simulink model "Project_2_2020a"  (R2020a)
settings: Solver=ode15s  StartTime=0.0  StopTime=10  MaxStep=0.2  RelTol=1e-2  EnableMultiTasking=on
model workspace (MAT data in the model file):
  g_density = 5
values from neighbouring files (symbols this model uses):
  Aa = 0    [execute_model_2020a.m]
  Ab = 0    [execute_model_2020a.m]
  Ac = 0    [execute_model_2020a.m]
  Ax = 0    [execute_model_2020a.m]
  Ay = 0    [execute_model_2020a.m]
  Az = 0    [execute_model_2020a.m]
  B = [24.233423136094 6.1219332628706 -6.1219332628706 -24.233423136094 -18.111489873223 18.111489873223 ... (first row only)    [execute_model_2020a.m]
  flange_len = 3    [execute_model_2020a.m]
  flange_thick = 0.8    [execute_model_2020a.m]
  flange_width = 2.25    [execute_model_2020a.m]
  hex_skew = -0.25    [execute_model_2020a.m]
  ka = 0    [execute_model_2020a.m]
  kb = 0    [execute_model_2020a.m]
  kc = 0    [execute_model_2020a.m]
  Kd = 8    [execute_model_2020a.m]
  Ki = 11.5    [execute_model_2020a.m]
  Kp = 450    [execute_model_2020a.m]
  kx = 0    [execute_model_2020a.m]
  ky = 0    [execute_model_2020a.m]
  kz = 75    [execute_model_2020a.m]
  leg_rad = 3    [execute_model_2020a.m]
  nom_length = 30    [execute_model_2020a.m]
  P = [14.574164873203 11.040422061358 -11.040422061358 -14.574164873203 -3.5337428118454 3.5337428118454 ... (first row only)    [execute_model_2020a.m]
  pa = 0    [execute_model_2020a.m]
  pb = 0    [execute_model_2020a.m]
  pc = 0    [execute_model_2020a.m]
  platform_rad = 18    [execute_model_2020a.m]
  platform_thick = 2    [execute_model_2020a.m]
  px = 0    [execute_model_2020a.m]
  py = 0    [execute_model_2020a.m]
  pz = 0    [execute_model_2020a.m]
  wa = 0    [execute_model_2020a.m]
  wb = 0    [execute_model_2020a.m]
  wc = 0    [execute_model_2020a.m]
  wx = 0    [execute_model_2020a.m]
  wy = 0    [execute_model_2020a.m]
  wz = 0    [execute_model_2020a.m]
undefined symbols (not defined in the file or in its folder): X, Y, Z
libraries: sm_stewart_platform_lib x13, sm_lib x10, nesl_utility x8, simulink x2, Parts_Lib x1, Contact_Forces_Lib x1, simulink_extras x1
(part 2 of 2)

== system Project_2_2020a/dy ==
  t : Inport
  Add : Sum  Inputs=|++
  Add2 : Sum  Inputs=++|
  amp1 : Gain  Gain=A
  amp2 : Gain  Gain=w*A*pi/180
  deg2rad : Gain  Gain=pi/180
  freq : Gain  Gain=w
  offset : Constant  Value=k  VectorParams1D=off
  phase : Constant  Value=p  VectorParams1D=off
  sin cos : Trigonometry  Operator=sincos
  f : Outport  VectorParamsAs1DForOutWhenUnconnected=off
  f' : Outport  Port=2  VectorParamsAs1DForOutWhenUnconnected=off
  wires:
  t/1 -> freq/1
  Add/1 -> deg2rad/1
  phase/1 -> Add/2
  amp2/1 -> f'/1
  Add2/1 -> f/1
  offset/1 -> Add2/1
  sin cos/1 -> amp1/1
  sin cos/2 -> amp2/1
  amp1/1 -> Add2/2
  freq/1 -> Add/1
  deg2rad/1 -> sin cos/1

== system Project_2_2020a/dz ==
  t : Inport
  Add : Sum  Inputs=|++
  Add2 : Sum  Inputs=++|
  amp1 : Gain  Gain=A
  amp2 : Gain  Gain=w*A*pi/180
  deg2rad : Gain  Gain=pi/180
  freq : Gain  Gain=w
  offset : Constant  Value=k  VectorParams1D=off
  phase : Constant  Value=p  VectorParams1D=off
  sin cos : Trigonometry  Operator=sincos
  f : Outport  VectorParamsAs1DForOutWhenUnconnected=off
  f' : Outport  Port=2  VectorParamsAs1DForOutWhenUnconnected=off
  wires:
  t/1 -> freq/1
  Add/1 -> deg2rad/1
  phase/1 -> Add/2
  amp2/1 -> f'/1
  Add2/1 -> f/1
  offset/1 -> Add2/1
  sin cos/1 -> amp1/1
  sin cos/2 -> amp2/1
  amp1/1 -> Add2/2
  freq/1 -> Add/1
  deg2rad/1 -> sin cos/1

== system Project_2_2020a/Euler XYZ Derivative/Skew Op ==
  v : Inport
  Demux : Demux  Outputs=3
  Demux1 : Demux  Outputs=3
  Gain : Gain  Gain=-1
  Mux6 : Mux  Inputs=9
  Reshape 9x1->3x3 : Reshape  OutputDimensionality=Customize  OutputDimensions=[3,3]
  Zero : Constant  Value=0
  v~ : Outport  VectorParamsAs1DForOutWhenUnconnected=off
  wires:
  Mux6/1 -> Reshape 9x1->3x3/1
  v/1 -> Demux/1, Gain/1
  Gain/1 -> Demux1/1
  Reshape 9x1->3x3/1 -> v~/1
  Zero/1 -> Mux6/1, Mux6/5, Mux6/9
  Demux/3 -> Mux6/2
  Demux1/2 -> Mux6/3
  Demux1/3 -> Mux6/4
  Demux/1 -> Mux6/6
  Demux/2 -> Mux6/7
  Demux1/1 -> Mux6/8

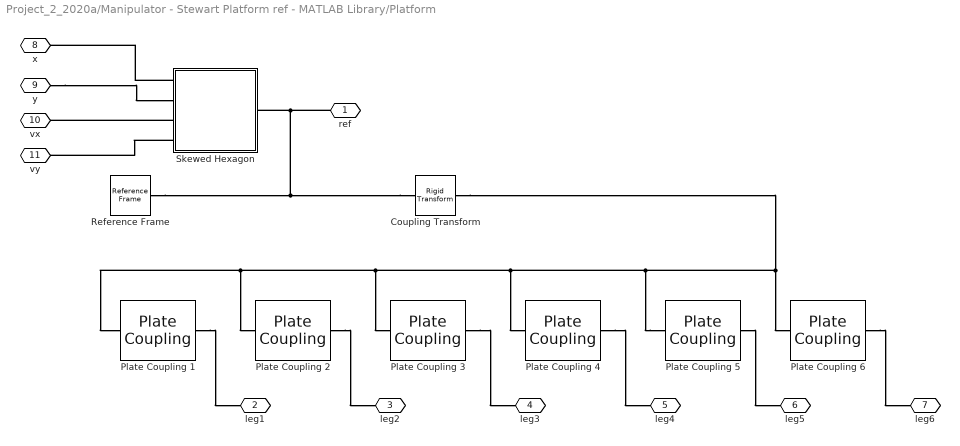
== system Project_2_2020a/Manipulator - Stewart Platform ref - MATLAB Library/Platform ==
  Coupling Transform : sm_lib/Frames and Transforms/Rigid Transform  TranslationMethod=StandardAxis  TranslationStandardOffset=(1 - 2 * kind_val) * (hex_thick / 2 + flange_len)  TranslationLengthUnit=cm  TranslationStandardAxis=+Z  TranslationCartesianOffset=[0 0 0]  TranslationROffset=0  TranslationROffsetUnits=m  TranslationZOffset=0  TranslationZOffsetUnits=m  TranslationThetaOffset=0  TranslationThetaOffsetUnits=deg  RotationMethod=AlignedAxes  RotationAngleUnits=deg  RotationStandardAxis=+Z  RotationAngle=0  RotationArbitraryAxis=[0 0 1]  FollAlignAxisA=+Z  BaseAlignAxisA=+X  FollAlignAxisB=+X  BaseAlignAxisB=+Z  RotationSequenceAxes=FollowerAxes  RotationSequence=XYX  RotationSequenceAngles=[0 0 0]  RotationSequenceAnglesUnits=deg  RotationMatrix=[1 0 0; 0 1 0; 0 0 1]  Quaternion=[1 0 0 0]
  Plate Coupling 1 : sm_stewart_platform_lib/Plate Coupling  index=0 + kind_val  hex_rad=hex_rad  hex_skew=hex_skew  flange_width=flange_width  flange_thick=flange_thick  flange_sep=flange_sep  flange_ref_rot=kind_val * 180
  Plate Coupling 2 : sm_stewart_platform_lib/Plate Coupling  index=1 + kind_val  hex_rad=hex_rad  hex_skew=hex_skew  flange_width=flange_width  flange_thick=flange_thick  flange_sep=flange_sep  flange_ref_rot=kind_val * 180
  Plate Coupling 3 : sm_stewart_platform_lib/Plate Coupling  index=2 + kind_val  hex_rad=hex_rad  hex_skew=hex_skew  flange_width=flange_width  flange_thick=flange_thick  flange_sep=flange_sep  flange_ref_rot=kind_val * 180
  Plate Coupling 4 : sm_stewart_platform_lib/Plate Coupling  index=3 + kind_val  hex_rad=hex_rad  hex_skew=hex_skew  flange_width=flange_width  flange_thick=flange_thick  flange_sep=flange_sep  flange_ref_rot=kind_val * 180
  Plate Coupling 5 : sm_stewart_platform_lib/Plate Coupling  index=4 + kind_val  hex_rad=hex_rad  hex_skew=hex_skew  flange_width=flange_width  flange_thick=flange_thick  flange_sep=flange_sep  flange_ref_rot=kind_val * 180
  Plate Coupling 6 : sm_stewart_platform_lib/Plate Coupling  index=mod(5 + kind_val, 6)  hex_rad=hex_rad  hex_skew=hex_skew  flange_width=flange_width  flange_thick=flange_thick  flange_sep=flange_sep  flange_ref_rot=kind_val * 180
  Reference Frame : sm_lib/Frames and Transforms/Reference Frame
  Skewed Hexagon : Subsystem  mask(Skewed Hexagon){rad=hex_rad, thick=hex_thick, skew=hex_skew, diffuse=diffuse, specualr=specular, shininess=shininess}
      mask prompts: rad "Radius (cm)"; thick "Thickness (cm)"; diffuse "Diffuse (rgba)"; specualr "Specular (rgba)"; shininess "Shininess (0-128)"
      mask help:
      | Models a hexagonal prism with 3-fold symmetry.
      |
      | A skew factor in the range (-0.5, +0.5) controls the shape of the hexagon.  A zero skew factor produces a regular hexagon cross section, and values toward +/- 0.5 produce progressively more triangular hexagons.
      mask init:
      | angles = pi/3 * ((0:1:5) + skew * [+1 -1 +1 -1 +1 -1]);
      | cross_sect = rad * [cos(angles); sin(angles)]';
      mask Help:
      | A <em>Skewed Hexagon</em> models a hexagonal prism with 3-fold symmetry.
      | 
      | A skew factor in the range (-0.5, +0.5) controls the shape of the hexagon.  A zero
      | skew factor produces a regular hexagon cross section, and values toward +/- 0.5
      | produce progressively more triangular hexagons.
      | 
      | See <em>Skewed Hexagons</em> in the documentation of the <em>Hexagon Plate</em>
      | block for more details.
      | 
      | <h3>Geometry</h3>
      | 
      | The <em>Geom</em> tab parameters specify the geometry of the skewed hexagon.
      | 
      | <ul>
      | 
      | <li> <b>Radius</b> The radius of thee circle on which the vertices of
      |   the hexagonal cross section lie.
      | 
      | <li> <b> Thickness</b> The thickness (length) of the hexagonal prism.
      | 
      | <li> <b>Skew</b> The skew factor of the hexagonal cross section, in the
      |   range (-0.5, +0.5).
      | 
      | </ul>
      | 
      | <h3>Visualization</h3>
      | 
      | The <em>Graphics</em> tab parameters specify the visualization aspects of the skewed
      | hexagon.
      | 
      | 
      | <ul>
      | 
      | <li> <b>Diffuse</b> The diffuse color of the skewed hexagon.  This is an RGB
      | 3-vector or an RGBA 4-vector with all components in the range [0, 1].
      | 
      | <li> <b>Specular</b> The specular color of the skewed hexagon.  This is an RGB
      | 3-vector or an RGBA 4-vector with all components in the range [0, 1].
      | 
      | <li> <b>Shininess</b> The shininess of the skewed hexagon.  This is a scalar
      | value in the range [0, 128].
      | 
      | </ul>
      | 
      | 
      | <h3>Ports</h3>
      | 
      | <ul>
      | 
      | <li> <b>ref</b> Reference frame of the skewed hexagon.  The origin of this frame
      |   is located at the center of the hexagonal prism, and the z-axis is aligned
      |   with the axis of the prism.
      | 
      | </ul>
      mask Display:
      | image('sm_stewart_platform_skewedhexagon.png')
      | color('white')
      | port_label('RConn', 1, 'ref')
  ref : PMIOPort  Side=Left
  leg1 : PMIOPort  Port=2  Side=Right
  leg2 : PMIOPort  Port=3  Side=Right
  leg3 : PMIOPort  Port=4  Side=Right
  leg4 : PMIOPort  Port=5  Side=Right
  leg5 : PMIOPort  Port=6  Side=Right
  leg6 : PMIOPort  Port=7  Side=Right
  x : PMIOPort  Port=8  Side=Left
  y : PMIOPort  Port=9  Side=Left
  vx : PMIOPort  Port=10  Side=Left
  vy : PMIOPort  Port=11  Side=Left
  connections:
  Plate Coupling 6/RConn1 -- leg6/RConn1
  Plate Coupling 5/RConn1 -- leg5/RConn1
  Plate Coupling 4/RConn1 -- leg4/RConn1
  Plate Coupling 3/RConn1 -- leg3/RConn1
  Plate Coupling 2/RConn1 -- leg2/RConn1
  Plate Coupling 1/RConn1 -- leg1/RConn1
  Plate Coupling 5/LConn1 -- Plate Coupling 4/LConn1 -- Plate Coupling 3/LConn1 -- Plate Coupling 1/LConn1 -- Plate Coupling 2/LConn1 -- Coupling Transform/RConn1 -- Plate Coupling 6/LConn1
  Coupling Transform/LConn1 -- ref/RConn1 -- Skewed Hexagon/RConn1 -- Reference Frame/RConn1
  Skewed Hexagon/LConn1 -- x/RConn1
  y/RConn1 -- Skewed Hexagon/LConn2
  Skewed Hexagon/LConn3 -- vx/RConn1
  Skewed Hexagon/LConn4 -- vy/RConn1

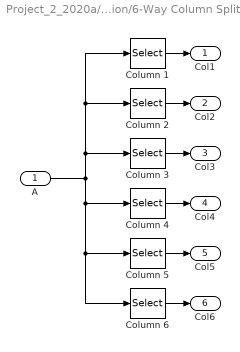
== system Project_2_2020a/Pos Computation/6-Way Column Splitter ==
  A : Inport
  Column 1 : Selector  NumberOfDimensions=2  InputPortWidth=3  IndexOptions=Select all,Index vector (dialog)  Indices=-1,1  OutputSizes=1
  Column 2 : Selector  NumberOfDimensions=2  InputPortWidth=3  IndexOptions=Select all,Index vector (dialog)  Indices=-1,2  OutputSizes=1
  Column 3 : Selector  NumberOfDimensions=2  InputPortWidth=3  IndexOptions=Select all,Index vector (dialog)  Indices=-1,3  OutputSizes=1
  Column 4 : Selector  NumberOfDimensions=2  InputPortWidth=3  IndexOptions=Select all,Index vector (dialog)  Indices=-1,4  OutputSizes=1
  Column 5 : Selector  NumberOfDimensions=2  InputPortWidth=3  IndexOptions=Select all,Index vector (dialog)  Indices=-1,5  OutputSizes=1
  Column 6 : Selector  NumberOfDimensions=2  InputPortWidth=3  IndexOptions=Select all,Index vector (dialog)  Indices=-1,6  OutputSizes=1
  Col1 : Outport  VectorParamsAs1DForOutWhenUnconnected=off
  Col2 : Outport  Port=2  VectorParamsAs1DForOutWhenUnconnected=off
  Col3 : Outport  Port=3  VectorParamsAs1DForOutWhenUnconnected=off
  Col4 : Outport  Port=4  VectorParamsAs1DForOutWhenUnconnected=off
  Col5 : Outport  Port=5  VectorParamsAs1DForOutWhenUnconnected=off
  Col6 : Outport  Port=6  VectorParamsAs1DForOutWhenUnconnected=off
  wires:
  A/1 -> Column 3/1, Column 2/1, Column 1/1, Column 4/1, Column 5/1, Column 6/1
  Column 1/1 -> Col1/1
  Column 2/1 -> Col2/1
  Column 3/1 -> Col3/1
  Column 4/1 -> Col4/1
  Column 5/1 -> Col5/1
  Column 6/1 -> Col6/1

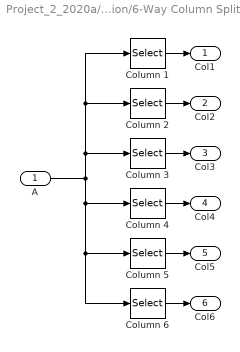
== system Project_2_2020a/Vel Computation/6-Way Column Splitter ==
  A : Inport
  Column 1 : Selector  NumberOfDimensions=2  InputPortWidth=3  IndexOptions=Select all,Index vector (dialog)  Indices=-1,1  OutputSizes=1
  Column 2 : Selector  NumberOfDimensions=2  InputPortWidth=3  IndexOptions=Select all,Index vector (dialog)  Indices=-1,2  OutputSizes=1
  Column 3 : Selector  NumberOfDimensions=2  InputPortWidth=3  IndexOptions=Select all,Index vector (dialog)  Indices=-1,3  OutputSizes=1
  Column 4 : Selector  NumberOfDimensions=2  InputPortWidth=3  IndexOptions=Select all,Index vector (dialog)  Indices=-1,4  OutputSizes=1
  Column 5 : Selector  NumberOfDimensions=2  InputPortWidth=3  IndexOptions=Select all,Index vector (dialog)  Indices=-1,5  OutputSizes=1
  Column 6 : Selector  NumberOfDimensions=2  InputPortWidth=3  IndexOptions=Select all,Index vector (dialog)  Indices=-1,6  OutputSizes=1
  Col1 : Outport  VectorParamsAs1DForOutWhenUnconnected=off
  Col2 : Outport  Port=2  VectorParamsAs1DForOutWhenUnconnected=off
  Col3 : Outport  Port=3  VectorParamsAs1DForOutWhenUnconnected=off
  Col4 : Outport  Port=4  VectorParamsAs1DForOutWhenUnconnected=off
  Col5 : Outport  Port=5  VectorParamsAs1DForOutWhenUnconnected=off
  Col6 : Outport  Port=6  VectorParamsAs1DForOutWhenUnconnected=off
  wires:
  A/1 -> Column 3/1, Column 2/1, Column 1/1, Column 4/1, Column 5/1, Column 6/1
  Column 1/1 -> Col1/1
  Column 2/1 -> Col2/1
  Column 3/1 -> Col3/1
  Column 4/1 -> Col4/1
  Column 5/1 -> Col5/1
  Column 6/1 -> Col6/1

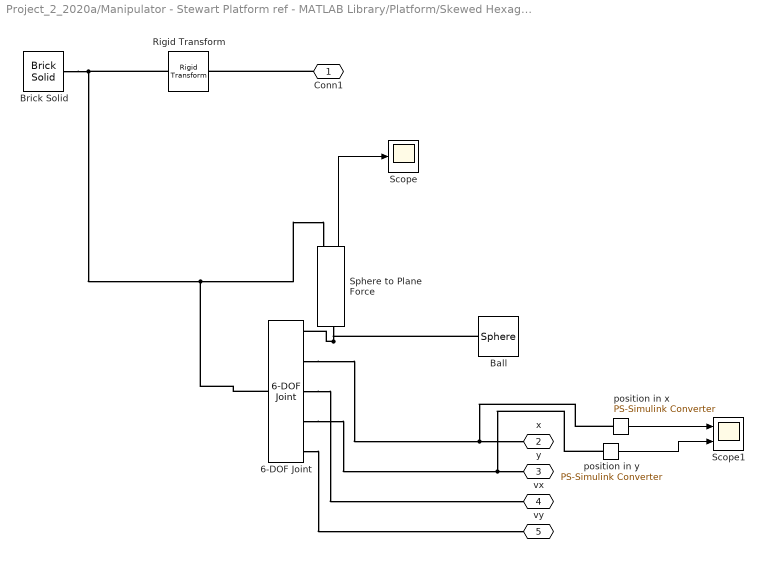
== system Project_2_2020a/Manipulator - Stewart Platform ref - MATLAB Library/Platform/Skewed Hexagon ==
  6-DOF Joint : sm_lib/Joints/6-DOF Joint  JointMode=Normal  SenseConstraintForce=off  SenseConstraintForceX=off  SenseConstraintForceY=off  SenseConstraintForceZ=off  SenseConstraintTorque=off  SenseConstraintTorqueX=off  SenseConstraintTorqueY=off  SenseConstraintTorqueZ=off  SenseTotalForce=off  SenseTotalForceX=off  SenseTotalForceY=off  SenseTotalForceZ=off  SenseTotalTorque=off  SenseTotalTorqueX=off  SenseTotalTorqueY=off  SenseTotalTorqueZ=off  CompositeWrenchDir=FollowerOnBase  CompositeWrenchFrame=BaseFrame  PxEquilibriumPosition=0  PxEquilibriumPositionUnits=m  PxSpringStiffness=0  PxSpringStiffnessUnits=N/m  PxDampingCoefficient=0  PxDampingCoefficientUnits=N/(m/s)  PxTorqueActuationMode=NoTorque  PxMotionActuationMode=ComputedMotion  PxSensePosition=on  PxSenseVelocity=on  PxSenseAcceleration=off  PxSenseTorqueForce=off  PxSenseLowerLimitTorqueForce=off  PxSenseUpperLimitTorqueForce=off  PxLowerLimitSpecify=off  PxLowerLimitBound=-1  PxLowerLimitBoundUnits=m  PxLowerLimitStiffness=1e6  PxLowerLimitStiffnessUnits=N/m  PxLowerLimitDamping=1e3  PxLowerLimitDampingUnits=N/(m/s)  PxLowerLimitTransitionRegionWidth=1e-4  PxLowerLimitTransitionRegionWidthUnits=m  PxUpperLimitSpecify=off  PxUpperLimitBound=1  PxUpperLimitBoundUnits=m  PxUpperLimitStiffness=1e6  PxUpperLimitStiffnessUnits=N/m  PxUpperLimitDamping=1e3  PxUpperLimitDampingUnits=N/(m/s)  PxUpperLimitTransitionRegionWidth=1e-4  PxUpperLimitTransitionRegionWidthUnits=m  PxPositionTargetSpecify=on  PxPositionTargetPriority=High  PxPositionTargetValue=0  PxPositionTargetValueUnits=m  PxVelocityTargetSpecify=on  PxVelocityTargetPriority=High  PxVelocityTargetValue=x_velocity  PxVelocityTargetValueUnits=m/s  PyEquilibriumPosition=0  PyEquilibriumPositionUnits=m  PySpringStiffness=0  PySpringStiffnessUnits=N/m  PyDampingCoefficient=0  PyDampingCoefficientUnits=N/(m/s)  PyTorqueActuationMode=NoTorque  PyMotionActuationMode=ComputedMotion  PySensePosition=on  PySenseVelocity=on  PySenseAcceleration=off  PySenseTorqueForce=off  PySenseLowerLimitTorqueForce=off  PySenseUpperLimitTorqueForce=off  PyLowerLimitSpecify=off  PyLowerLimitBound=-1  PyLowerLimitBoundUnits=m  PyLowerLimitStiffness=1e6  PyLowerLimitStiffnessUnits=N/m  PyLowerLimitDamping=1e3  PyLowerLimitDampingUnits=N/(m/s)  PyLowerLimitTransitionRegionWidth=1e-4  PyLowerLimitTransitionRegionWidthUnits=m  PyUpperLimitSpecify=off  PyUpperLimitBound=1  PyUpperLimitBoundUnits=m  PyUpperLimitStiffness=1e6  PyUpperLimitStiffnessUnits=N/m  PyUpperLimitDamping=1e3  PyUpperLimitDampingUnits=N/(m/s)  PyUpperLimitTransitionRegionWidth=1e-4  PyUpperLimitTransitionRegionWidthUnits=m  PyPositionTargetSpecify=on  PyPositionTargetPriority=High  PyPositionTargetValue=0  PyPositionTargetValueUnits=m  PyVelocityTargetSpecify=on  PyVelocityTargetPriority=High  PyVelocityTargetValue=y_velocity  PyVelocityTargetValueUnits=m/s  PzEquilibriumPosition=0  PzEquilibriumPositionUnits=m  PzSpringStiffness=0  PzSpringStiffnessUnits=N/m  PzDampingCoefficient=0  PzDampingCoefficientUnits=N/(m/s)  PzTorqueActuationMode=NoTorque  PzMotionActuationMode=ComputedMotion  PzSensePosition=off  PzSenseVelocity=off  PzSenseAcceleration=off  PzSenseTorqueForce=off  PzSenseLowerLimitTorqueForce=off  PzSenseUpperLimitTorqueForce=off  PzLowerLimitSpecify=off  PzLowerLimitBound=-1  PzLowerLimitBoundUnits=m  PzLowerLimitStiffness=1e6  PzLowerLimitStiffnessUnits=N/m  PzLowerLimitDamping=1e3  PzLowerLimitDampingUnits=N/(m/s)  PzLowerLimitTransitionRegionWidth=1e-4  PzLowerLimitTransitionRegionWidthUnits=m  PzUpperLimitSpecify=off  PzUpperLimitBound=1  PzUpperLimitBoundUnits=m  PzUpperLimitStiffness=1e6  PzUpperLimitStiffnessUnits=N/m  PzUpperLimitDamping=1e3  PzUpperLimitDampingUnits=N/(m/s)  PzUpperLimitTransitionRegionWidth=1e-4  PzUpperLimitTransitionRegionWidthUnits=m  PzPositionTargetSpecify=on  PzPositionTargetPriority=High  PzPositionTargetValue=0.03+0.2  PzPositionTargetValueUnits=m  PzVelocityTargetSpecify=on  PzVelocityTargetPriority=High  PzVelocityTargetValue=0  PzVelocityTargetValueUnits=m/s  SphEqPosRotationMethod=None  SphEqPosRotationAngleUnits=deg  SphEqPosRotationStandardAxis=+Z  SphEqPosRotationAngle=0.0  SphEqPosRotationArbitraryAxis=[0 0 1]  SphEqPosFollAlignAxisA=+X  SphEqPosBaseAlignAxisA=+Y  SphEqPosFollAlignAxisB=+Y  SphEqPosBaseAlignAxisB=+Z  SphEqPosRotationSequenceAxes=FollowerAxes  SphEqPosRotationSequence=XYX  SphEqPosRotationSequenceAngles=[0 0 0]  SphEqPosRotationSequenceAnglesUnits=deg  SphEqPosRotationMatrix=[1 0 0; 0 1 0; 0 0 1]  SphEqPosQuaternion=[1 0 0 0]  SphSpringStiffness=0  SphSpringStiffnessUnits=N*m/deg  SphDampingCoefficient=0  SphDampingCoefficientUnits=N*m/(deg/s)  SphActuateTorqueX=off  SphActuateTorqueY=off  SphActuateTorqueZ=off  SphActuateTorque=off  SphTorqueActuationMode=NoTorque  SphMotionActuationMode=ComputedMotion  SphActuationFrame=BaseFrame  SphSensePosition=off  SphSenseVelocityX=off  SphSenseVelocityY=off  SphSenseVelocityZ=off  SphSenseVelocity=off  SphSenseAccelerationX=off  SphSenseAccelerationY=off  SphSenseAccelerationZ=off  SphSenseAcceleration=off  SphSenseTorqueX=off  SphSenseTorqueY=off  SphSenseTorqueZ=off  SphSenseTorqueForce=off  SphSenseLowerLimitTorqueMag=off  SphSenseUpperLimitTorqueMag=off  SphSensingFrame=BaseFrame  SphLowerLimitSpecify=off  SphLowerLimitBound=15  SphLowerLimitBoundUnits=deg  SphLowerLimitStiffness=1e4  SphLowerLimitStiffnessUnits=N*m/deg  SphLowerLimitDamping=10  SphLowerLimitDampingUnits=N*m/(deg/s)  SphLowerLimitTransitionRegionWidth=0.1  SphLowerLimitTransitionRegionWidthUnits=deg  SphUpperLimitSpecify=off  SphUpperLimitBound=45  SphUpperLimitBoundUnits=deg  SphUpperLimitStiffness=1e4  SphUpperLimitStiffnessUnits=N*m/deg  SphUpperLimitDamping=10  SphUpperLimitDampingUnits=N*m/(deg/s)  SphUpperLimitTransitionRegionWidth=0.1  SphUpperLimitTransitionRegionWidthUnits=deg  SphPositionTargetRotationMethod=None  SphPositionTargetRotationAngleUnits=deg  SphPositionTargetRotationStandardAxis=+Z  SphPositionTargetRotationAngle=0.0  SphPositionTargetRotationArbitraryAxis=[0 0 1]  SphPositionTargetFollAlignAxisA=+X  SphPositionTargetBaseAlignAxisA=+Y  SphPositionTargetFollAlignAxisB=+Y  SphPositionTargetBaseAlignAxisB=+Z  SphPositionTargetRotationSequenceAxes=FollowerAxes  SphPositionTargetRotationSequence=XYX  SphPositionTargetRotationSequenceAngles=[0 0 0]  SphPositionTargetRotationSequenceAnglesUnits=deg  SphPositionTargetRotationMatrix=[1 0 0; 0 1 0; 0 0 1]  SphPositionTargetQuaternion=[1 0 0 0]  SphPositionTargetSpecify=off  SphPositionTargetPriority=High  SphVelocityTargetValue=[0 0 0]  SphVelocityTargetValueUnits=deg/s  SphVelocityTargetSpecify=on  SphVelocityTargetPriority=High  SphVelocityTargetInFollowerFrame=on
  Ball : Parts_Lib/Sphere  Tag=CustomStyle  sph_radius=0.02  sph_density=5000  sph_color=gray  sph_opacity=1  mark_type=Rings on center planes  arc_width=[40 50]  arc_angle=60  ring_width=5  ring_irad=0.95  mark_color=axes  mark_opacity_x=1  mark_opacity_y=1  mark_opacity_z=1  mark_opacity=1  ring_opacity=0  arc_opacity=0  arc_extr_data=0
  Brick Solid : sm_lib/Body Elements/Brick Solid  GraphicAmbientColor=[0.15 0.15 0.15 1.0]  BasedOnType=Density  BrickDimensions=[70 70 4]  BrickDimensionUnits=cm  CenterOfMass=[0 0 0]  CenterOfMassUnits=m  GraphicDiffuseColor=[0.8 0.6 0.7]  Density=1000  DensityUnits=kg/m^3  DoExposeReferenceFrame=on  GraphicEmissiveColor=[0.0 0.0 0.0 1.0]  ExportEntireGeometry=off  SerializedFrames=<Frames/>  MarkerShape=Sphere  MarkerSize=10  GraphicType=FromGeometry  InertiaType=CalculateFromGeometry  Mass=1  MassUnits=kg  MomentsOfInertia=[1 1 1]  MomentsOfInertiaUnits=kg*m^2  GraphicOpacity=1  ProductsOfInertia=[0 0 0]  ProductsOfInertiaUnits=kg*m^2  GraphicShininess=75  GraphicSpecularColor=[0.5 0.5 0.5 1.0]  GraphicVisPropType=SimpleVisualProperties
  Rigid Transform : sm_lib/Frames and Transforms/Rigid Transform  TranslationMethod=None  TranslationStandardOffset=0  TranslationLengthUnit=m  TranslationStandardAxis=+Z  TranslationCartesianOffset=[0 0 0]  TranslationROffset=0  TranslationROffsetUnits=m  TranslationZOffset=0  TranslationZOffsetUnits=m  TranslationThetaOffset=0  TranslationThetaOffsetUnits=deg  RotationMethod=StandardAxis  RotationAngleUnits=deg  RotationStandardAxis=+Z  RotationAngle=60  RotationArbitraryAxis=[0 0 1]  FollAlignAxisA=+X  BaseAlignAxisA=+Y  FollAlignAxisB=+Y  BaseAlignAxisB=+Z  RotationSequenceAxes=FollowerAxes  RotationSequence=XYX  RotationSequenceAngles=[0 0 0]  RotationSequenceAnglesUnits=deg  RotationMatrix=[1 0 0; 0 1 0; 0 0 1]  Quaternion=[1 0 0 0]
  Scope : Scope
  Scope1 : Scope  NumInputPorts=2
  Sphere to Plane Force : Contact_Forces_Lib/3D/Sphere to Plane Force  sphere_rad=0.02  plane_lenx=0.70  plane_leny=0.70  plane_depth=0.02  force_law=Linear  k_contact=1000  b_contact=50  pen_full_damp_F=1e-4  pen_exponent=1  custom_param_1=1  custom_param_2=1  friction_law=Stick-Slip Continuous  mu_kinetic=0.9  mu_static=0.95  v_thr=1e-4  vis_on=on  vis_opc_en=0  vis_len_plaBz=0.005  vis_clr=[0.9 0.2 0.2]  vis_opc=0
  position in x : nesl_utility/PS-Simulink Converter  PhysicalDomain=network_engine_domain  SubClassName=ps_output  LeftPortType=input  RightPortType=output  PseudoPeriodic=off  Frequencies=[]  VectorFormat=inherit  Unit=inherit  AffineConversion=off
  "position in y " : nesl_utility/PS-Simulink Converter  PhysicalDomain=network_engine_domain  SubClassName=ps_output  LeftPortType=input  RightPortType=output  PseudoPeriodic=off  Frequencies=[]  VectorFormat=inherit  Unit=inherit  AffineConversion=off
  Conn1 : PMIOPort  Side=Right
  x : PMIOPort  Port=2  Side=Left
  y : PMIOPort  Port=3  Side=Left
  vx : PMIOPort  Port=4  Side=Left
  vy : PMIOPort  Port=5  Side=Left
  wires:
  Sphere to Plane Force/1 -> Scope/1
  position in x/1 -> Scope1/1
  "position in y "/1 -> Scope1/2
  connections:
  Ball/LConn1 -- Sphere to Plane Force/LConn1 -- 6-DOF Joint/RConn1
  Brick Solid/RConn1 -- Rigid Transform/RConn1 -- 6-DOF Joint/LConn1 -- Sphere to Plane Force/RConn1
  Conn1/RConn1 -- Rigid Transform/LConn1
  6-DOF Joint/RConn2 -- position in x/LConn1 -- x/RConn1
  6-DOF Joint/RConn3 -- vx/RConn1
  6-DOF Joint/RConn4 -- "position in y "/LConn1 -- y/RConn1
  6-DOF Joint/RConn5 -- vy/RConn1
